simulink model "Hbridge"  (R2021a)
settings: Solver=VariableStepAuto  StartTime=0.0  StopTime=10.0  RelTol=1e-3
libraries: spsSeriesRLCBranchLib x4, spsIGBTDiodeLib x2, spsVoltageMeasurementLib x2, spsCurrentMeasurementLib x1, spsDCVoltageSourceLib x1, spspowerguiLib x1
settings Model: Creator=Asus  LastModifiedBy=User

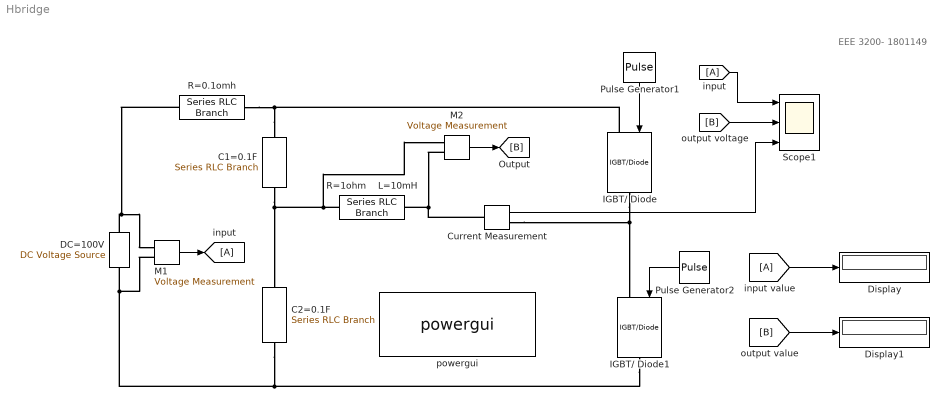
== system Hbridge ==
  note: EEE 3200- 1801149
  C1=0.1F : spsSeriesRLCBranchLib/Series RLC Branch  LConnTagsString=__new0  RConnTagsString=__new0  BranchType=C  Resistance=1  Inductance=19.53e-6  SetiL0=off  InitialCurrent=0  Capacitance=100000e-6  Setx0=off  InitialVoltage=0  Measurements=None
  "C2=0.1F  " : spsSeriesRLCBranchLib/Series RLC Branch  LConnTagsString=__new0  RConnTagsString=__new0  BranchType=C  Resistance=1  Inductance=19.53e-6  SetiL0=off  InitialCurrent=0  Capacitance=100000e-6  Setx0=off  InitialVoltage=0  Measurements=None
  Current Measurement : spsCurrentMeasurementLib/Current Measurement  PhasorSimulation=off  OutputType=Complex  PSBequivalent=0
  "DC=100V " : spsDCVoltageSourceLib/DC Voltage Source  Amplitude=100  Measurements=None
  Display : Display
  Display1 : Display
  IGBT/ Diode : spsIGBTDiodeLib/IGBT//Diode  Ron=1e-3  Rs=1e5  Cs=inf  Measurements=off
  IGBT/ Diode1 : spsIGBTDiodeLib/IGBT//Diode  Ron=1e-3  Rs=1e5  Cs=inf  Measurements=off
  M1 : spsVoltageMeasurementLib/Voltage Measurement  PhasorSimulation=off  OutputType=Complex  PSBequivalent=0
  M2 : spsVoltageMeasurementLib/Voltage Measurement  PhasorSimulation=off  OutputType=Complex  PSBequivalent=0
  Pulse Generator1 : DiscretePulseGenerator  PulseType=Time based  Period=.02  PulseWidth=50
  Pulse Generator2 : DiscretePulseGenerator  PulseType=Time based  Period=.02  PulseWidth=50  PhaseDelay=.01
  R=0.1omh : spsSeriesRLCBranchLib/Series RLC Branch  LConnTagsString=__new0  RConnTagsString=__new0  BranchType=R  Resistance=0.1  Inductance=25e-3  SetiL0=off  InitialCurrent=0  Capacitance=1e-6  Setx0=off  InitialVoltage=0  Measurements=None
  R=1ohm    L=10mH : spsSeriesRLCBranchLib/Series RLC Branch  LConnTagsString=__new0  RConnTagsString=__new0  BranchType=RL  Resistance=1  Inductance=10e-3  SetiL0=off  InitialCurrent=0  Capacitance=1e-6  Setx0=off  InitialVoltage=0  Measurements=None
  Scope1 : Scope  NumInputPorts=3
  powergui : spspowerguiLib/powergui  Priority=1  SimulationMode=Discrete  SampleTime=50e-6  frequency=60  Iterations=50  frequencyindice=0  Pbase=100e6  ErrMax=1e-4  UnitsV=kV  UnitsW=MW  buscounter=0  FunctionMessages=off  echomessages=off  EnableUseOfTLC=off  CurrentSourceSwitches=off  DisableSnubberDevices=off  DisableRonSwitches=off  DisableVfSwitches=off  DisplayEquations=off  AutomaticDiscreteSolvers=off  SolverType=Tustin/Backward Euler (TBE)  Interpol=off  ExternalGateDelay=off  methode=off  Ts=10  x0status=blocks  SPID=off  SwTol=0  HookPort=off  NonlinearTolerance=1e-4  nMaxIteration=100  ContinueOnMaxIteration=off  RestoreLinks=warning  ResistiveCurrentMeasurement=off  Frange=[0:2:500]  Ylog=off  Xlog=on  ShowGrid=off  save=off  variable=ZData  structure=0  ZoomFFT=off  StartTime=0.0  cycles=1  DisplayStyle=1  fundamental=60  FreqAxis=off  MaxFrequency=1000  frequencyindicesteady=1  RmsSteady=1  display=off
  wires:
  M2/1 -> [B]
  Pulse Generator2/1 -> IGBT/ Diode1/1
  Pulse Generator1/1 -> IGBT/ Diode/1
  [B] -> Display1/1
  [A] -> Display/1
  [A] -> Scope1/1
  Current Measurement/1 -> Scope1/3
  [B] -> Scope1/2
  M1/1 -> [A]
  connections:
  C1=0.1F/LConn1 -- IGBT/ Diode/LConn1 -- R=0.1omh/RConn1
  R=1ohm    L=10mH/RConn1 -- M2/LConn1 -- Current Measurement/LConn1
  R=1ohm    L=10mH/LConn1 -- M2/LConn2 -- C1=0.1F/RConn1 -- "C2=0.1F  "/LConn1
  IGBT/ Diode1/RConn1 -- M1/LConn2 -- "DC=100V "/LConn1 -- "C2=0.1F  "/RConn1
  Current Measurement/RConn1 -- IGBT/ Diode/RConn1 -- IGBT/ Diode1/LConn1
  M1/LConn1 -- "DC=100V "/RConn1 -- R=0.1omh/LConn1
